simulink model "reaction_wheel_array"  (R2015a)
settings: Solver=FixedStepDiscrete  StartTime=0.0  StopTime=10.0  FixedStep=delta_t  RelTol=1e-3
undefined symbols (not defined in the file): D, S
settings Model: Creator=Kerianne  LastModifiedBy=Kerianne
settings DataIOCC: SaveFormat=Structure
settings OptimizationCC: InlineParams=on  ExpressionDepthLimit=2147483647
settings DebuggingCC: UnderspecifiedInitializationDetection=Classic  MergeDetectMultiDrivingBlocksExec=none  SolverPrmCheckMsg=warning  StateNameClashWarn=warning

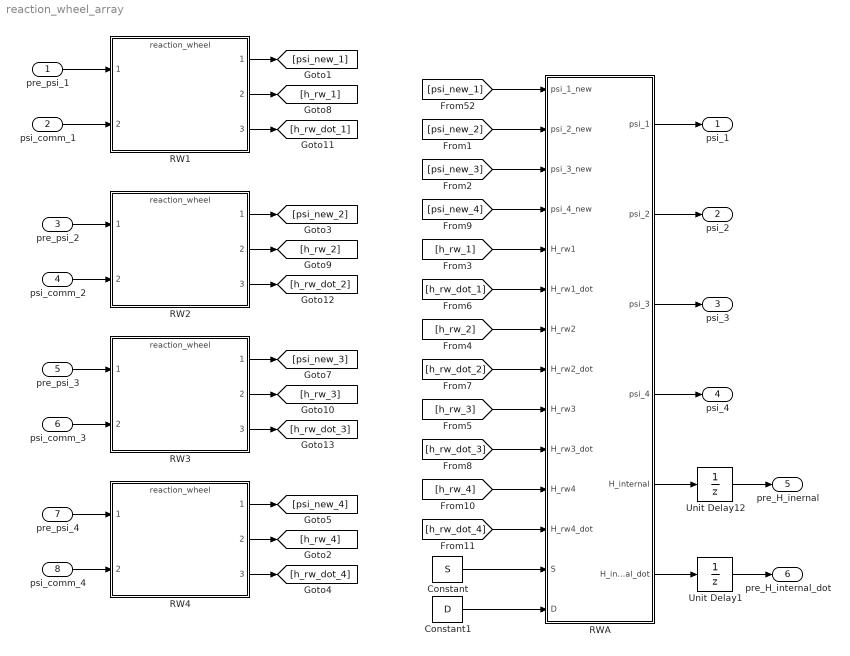
== system reaction_wheel_array ==
  pre_psi_1 : Inport
  "psi_comm_1 " : Inport  Port=2
  pre_psi_2 : Inport  Port=3
  psi_comm_2 : Inport  Port=4
  pre_psi_3 : Inport  Port=5
  psi_comm_3 : Inport  Port=6
  pre_psi_4 : Inport  Port=7
  psi_comm_4 : Inport  Port=8
  Constant : Constant  Value=S
  Constant1 : Constant  Value=D
  RW{1..4} (4 alike) : ModelReference  ModelNameDialog=reaction_wheel  SimulationMode=Normal  ModelReferenceVersion=1.5  CopyOfModelName=reaction_wheel  DefaultDataLogging=on
  RWA : MATLAB Function  TreatAsAtomicUnit=on
  Unit Delay1 : UnitDelay  InitialCondition=[0;0;0]  SampleTime=-1
  Unit Delay12 : UnitDelay  InitialCondition=[0;0;0]  SampleTime=-1
  psi_1 : Outport
  psi_2 : Outport  Port=2
  psi_3 : Outport  Port=3
  psi_4 : Outport  Port=4
  pre_H_inernal : Outport  Port=5  PortDimensions=3
  pre_H_internal_dot : Outport  Port=6  PortDimensions=3
  wires:
  RWA/1(psi_1) -> psi_1/1
  RWA/2(psi_2) -> psi_2/1
  RWA/3(psi_3) -> psi_3/1
  RWA/5(H_internal) -> Unit Delay12/1
  RWA/6(H_internal_dot) -> Unit Delay1/1
  Unit Delay12/1 -> pre_H_inernal/1
  [psi_new_2] -> RWA/2(psi_2_new)
  [psi_new_1] -> RWA/1(psi_1_new)
  pre_psi_1/1 -> RW1/1
  "psi_comm_1 "/1 -> RW1/2
  pre_psi_3/1 -> RW3/1
  psi_comm_3/1 -> RW3/2
  pre_psi_2/1 -> RW2/1
  psi_comm_2/1 -> RW2/2
  RW3/1 -> [psi_new_3]
  RW2/1 -> [psi_new_2]
  RW1/1 -> [psi_new_1]
  RW3/3 -> [h_rw_dot_3]
  RW3/2 -> [h_rw_3]
  RW2/2 -> [h_rw_2]
  RW2/3 -> [h_rw_dot_2]
  RW1/2 -> [h_rw_1]
  RW1/3 -> [h_rw_dot_1]
  [psi_new_3] -> RWA/3(psi_3_new)
  [h_rw_dot_3] -> RWA/10(H_rw3_dot)
  [h_rw_3] -> RWA/9(H_rw3)
  [h_rw_dot_2] -> RWA/8(H_rw2_dot)
  [h_rw_2] -> RWA/7(H_rw2)
  [h_rw_dot_1] -> RWA/6(H_rw1_dot)
  [h_rw_1] -> RWA/5(H_rw1)
  Unit Delay1/1 -> pre_H_internal_dot/1
  pre_psi_4/1 -> RW4/1
  psi_comm_4/1 -> RW4/2
  RW4/1 -> [psi_new_4]
  RW4/3 -> [h_rw_dot_4]
  RW4/2 -> [h_rw_4]
  [psi_new_4] -> RWA/4(psi_4_new)
  [h_rw_dot_4] -> RWA/12(H_rw4_dot)
  [h_rw_4] -> RWA/11(H_rw4)
  Constant/1 -> RWA/13(S)
  RWA/4(psi_4) -> psi_4/1
  Constant1/1 -> RWA/14(D)

== matlab function reaction_wheel_array/RWA ==
  data: psi_1_new input; psi_2_new input; psi_3_new input; psi_4_new input; psi_1 output; psi_2 output; psi_3 output; psi_4 output; H_rw1 input; H_rw1_dot input; H_rw2 input; H_rw2_dot input; H_rw3 input; H_rw3_dot input; H_internal output; H_internal_dot output; H_rw4 input; H_rw4_dot input; S input; D input
function [psi_1,psi_2,psi_3,psi_4,H_internal,H_internal_dot]= fcn(psi_1_new,psi_2_new,psi_3_new,psi_4_new,H_rw1,H_rw1_dot,H_rw2,H_rw2_dot,H_rw3,H_rw3_dot,H_rw4,H_rw4_dot,S,D)
% Reaction Wheel Array Simulation
% Author: Kerianne Gross, AFRL/RQQA, kerianne.gross@us.af.mil
% Last Updated: 7 May 2015 

% The sole purpose of the reaction wheel array block is to orient the
% angular momentum with the body frame

% "Hall sensor" output of angular rates
psi_1= psi_1_new;
psi_2= psi_2_new;
psi_3= psi_3_new;
psi_4= psi_4_new;

% Angular Momentum
H_internal = (1/D)*S*[H_rw1;H_rw2;H_rw3;H_rw4];   
% Change in Angular Momentum
H_internal_dot = (1/D)*S*[H_rw1_dot;H_rw2_dot;H_rw3_dot;H_rw4_dot];
